simulink subsystem "ideal_heatsrc"  (R2022b)
settings: Solver=VariableStepAuto  StartTime=0.0  StopTime=10.0  RelTol=1e-3
undefined symbols (not defined in the file or in its folder): flame
libraries: fl_lib x5, nesl_utility x1
settings Model: Creator=wilde  LastModifiedBy=wilde

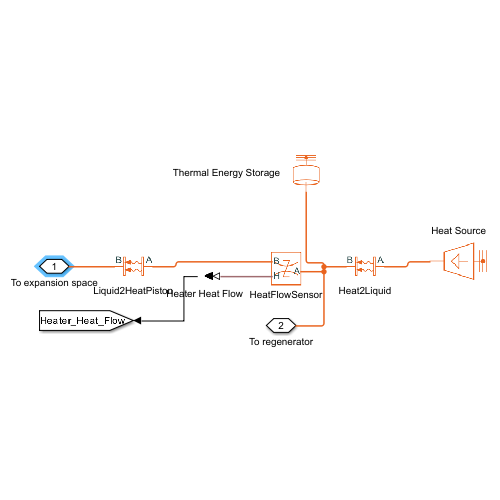
[thumbnail: Simulink's stored preview of the top-level diagram]
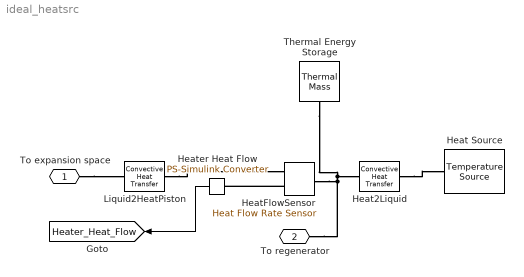
== system ideal_heatsrc ==
  Heat Source : fl_lib/Thermal/Thermal Sources/Temperature Source  temperature=flame.temperature K
  Heat2Liquid : fl_lib/Thermal/Thermal Elements/Convective Heat Transfer  thermal_type=foundation.enum.constant_variable.constant  area=f.flame.glass.area m^2  heat_tr_coeff=f.glass.gas.h W/(K*m^2)  min_heat_tr_coeff=1e-3 W/(K*m^2)  T_specify=off  T_priority=None  T=0 K  T_nominal_specify=off  T_nominal_unit=K  T_nominal_value=1  Q_specify=off  Q_priority=Low  Q=1e3 W  Q_nominal_specify=off  Q_nominal_unit=W  Q_nominal_value=1
  HeatFlowSensor : fl_lib/Thermal/Thermal Sensors/Heat Flow Rate Sensor
  Heater Heat Flow : nesl_utility/PS-Simulink Converter  PhysicalDomain=network_engine_domain  SubClassName=ps_output  LeftPortType=input  RightPortType=output  PseudoPeriodic=off  Frequencies=[]  VectorFormat=inherit  Unit=inherit  AffineConversion=off
  Liquid2HeatPiston : fl_lib/Thermal/Thermal Elements/Convective Heat Transfer  thermal_type=foundation.enum.constant_variable.constant  area=f.flame.glass.area m^2  heat_tr_coeff=f.glass.gas.h W/(K*m^2)  min_heat_tr_coeff=1e-3 W/(K*m^2)  T_specify=off  T_priority=None  T=0 K  T_nominal_specify=off  T_nominal_unit=K  T_nominal_value=1  Q_specify=off  Q_priority=None  Q=0 W  Q_nominal_specify=off  Q_nominal_unit=W  Q_nominal_value=1
  Thermal Energy Storage : fl_lib/Thermal/Thermal Elements/Thermal Mass  mass=flame.glass.m kg  sp_heat=flame.glass.cp J/(K*kg)  num_ports=foundation.enum.numPorts2.one  T_specify=on  T_priority=High  T=flame.glass.T.init K  T_nominal_specify=off  T_nominal_unit=K  T_nominal_value=1  Q_specify=off  Q_priority=None  Q=0 W  Q_nominal_specify=off  Q_nominal_unit=W  Q_nominal_value=1
  To expansion space : PMIOPort  Side=Left
  To regenerator : PMIOPort  Port=2  Side=Left
  tag scope: Heater_Heat_Flow=global
  wires:
  Heater Heat Flow/1 -> [Heater_Heat_Flow]
  connections:
  HeatFlowSensor/LConn1 -- To regenerator/RConn1 -- Heat2Liquid/RConn1 -- Thermal Energy Storage/LConn1
  Heat2Liquid/LConn1 -- Heat Source/LConn1
  To expansion space/RConn1 -- Liquid2HeatPiston/RConn1
  Liquid2HeatPiston/LConn1 -- HeatFlowSensor/RConn2
  HeatFlowSensor/RConn1 -- Heater Heat Flow/LConn1
